simulink model "HyperloopAED"  (R2025b)
settings: Solver=VariableStepAuto  StartTime=0.0  StopTime=30  RelTol=1e-3
settings Model: Creator=PRANAV  LastModifiedBy=PRANAV

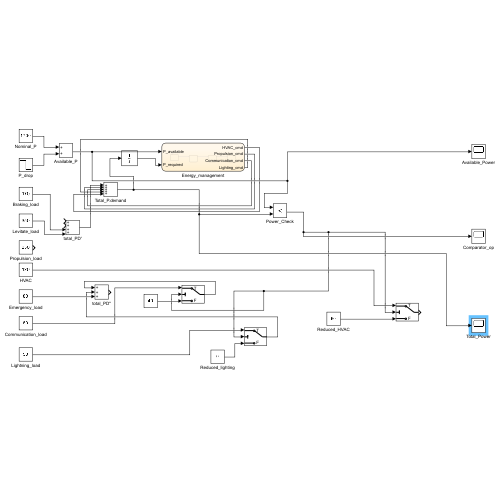
[thumbnail: Simulink's stored preview of the top-level diagram]
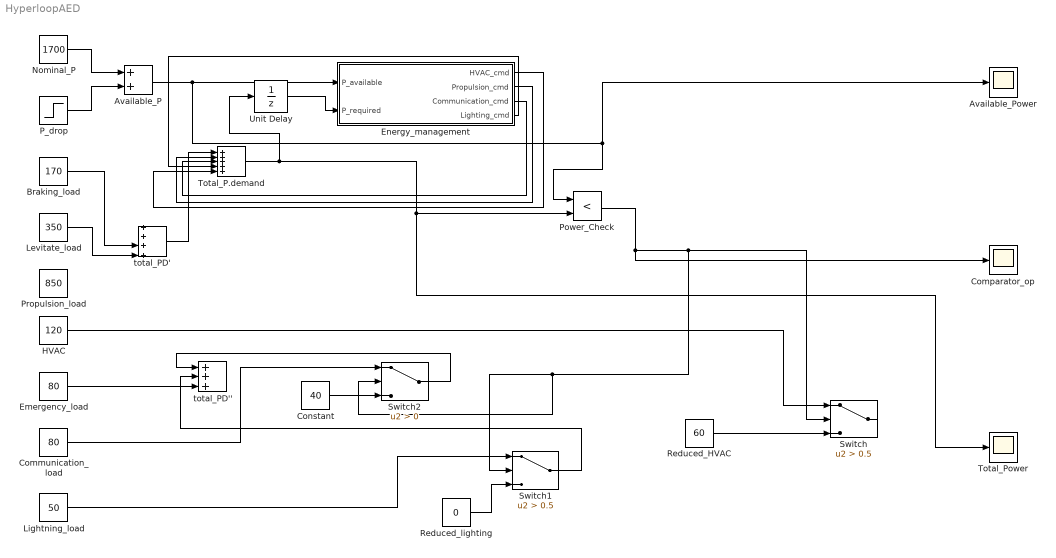
== system HyperloopAED ==
  Available_P : Sum
  Available_Power : Scope
      settings: ActiveDisplayYMinimum=1137.5  ActiveDisplayYMaximum=1762.5
  Braking_load : Constant  Value=170
  Communication_load : Constant  Value=80
  Comparator_op : Scope
      settings: ActiveDisplayYMinimum=-0.12499999999999997  ActiveDisplayYMaximum=1.125
  Constant : Constant  Value=40
  Emergency_load : Constant  Value=80
  Energy_management : Stateflow chart  TreatAsAtomicUnit=on
      settings: PortSchema="{\"entries\":[{\"content\":{\"sides\":[{\"content\":{\"connectorIds\":[\"In1\",\"In2\"]},\"type\":\"ConnectorPlacement.EquallySpacedRectSide\",\"uuid\":\"97038daa-e770-4b03-9197-b8205fec80ee\"},{\"content\":{\"connectorIds\":[\"Out1\",\"Out4\",\"Out3\",\"Out2\"],\"side\":\"RIGHT\"},\"type\":\"ConnectorPlacement.EquallySpacedRectSide\",\"uuid\":\"5d348c5e-e4cd-48d6-bfb1-b7eca039e31a\"},{\"content\":{\"side\":\"TOP\"},\"type\":\"ConnectorPlacement.EquallySpacedRectSide\",\"uuid\":\"902d5b1e-b622-43c9-be24-94d491fd9ea6\"}]},\"type\":\"ConnectorPlacement.EquallySpacedConnector\",\"uuid\":\"16dbb211-ee92-4295-a02a-abd65ddea233\"}],\"packageUris\":[\"http://schema.mathworks.com/mf0/Connector/R2020b\"],\"version\":\"1.0\"}"
  HVAC : Constant  Value=120
  Levitate_load : Constant  Value=350
  Lightning_load : Constant  Value=50
  Nominal_P : Constant  Value=1700
  P_drop : Step  Time=20  After=-500  SampleTime=0
  Power_Check : RelationalOperator  Operator=<  OutDataTypeStr=boolean  RndMeth=Simplest  InputSameDT=off
  Propulsion_load : Constant  Value=850
  Reduced_HVAC : Constant  Value=60
  Reduced_lighting : Constant  Value=0
  Switch : Switch  Criteria=u2 > Threshold  Threshold=0.5  SaturateOnIntegerOverflow=off  InputSameDT=off
  Switch1 : Switch  Criteria=u2 > Threshold  Threshold=0.5  SaturateOnIntegerOverflow=off  InputSameDT=off
  Switch2 : Switch  Criteria=u2 > Threshold  SaturateOnIntegerOverflow=off  InputSameDT=off
  Total_P.demand : Sum  Inputs=+++++
  Total_Power : Scope
      settings: ActiveDisplayYMinimum=965.125219697243  ActiveDisplayYMaximum=2457.5560129704977  DataLoggingVariableName=ScopeData2
  Unit Delay : UnitDelay  InitialCondition=1700  SampleTime=-1  HasFrameUpgradeWarning=on
  total_PD' : Sum  Inputs=++++
  total_PD'' : Sum  Inputs=+++
  wires:
  Nominal_P/1 -> Available_P/1
  P_drop/1 -> Available_P/2
  Levitate_load/1 -> total_PD'/4
  Braking_load/1 -> total_PD'/3
  Emergency_load/1 -> total_PD''/3
  total_PD'/1 -> Total_P.demand/1
  Available_P/1 -> Power_Check/1, Available_Power/1, Energy_management/1(P_available)
  Total_P.demand/1 -> Unit Delay/1, Total_Power/1, Power_Check/2
  Power_Check/1 -> Comparator_op/1, Switch2/2, Switch1/2, Switch/2
  HVAC/1 -> Switch/1
  Reduced_HVAC/1 -> Switch/3
  Lightning_load/1 -> Switch1/1
  Reduced_lighting/1 -> Switch1/3
  Switch1/1 -> total_PD''/2
  Constant/1 -> Switch2/3
  Communication_load/1 -> Switch2/1
  Switch2/1 -> total_PD''/1
  Energy_management/1(HVAC_cmd) -> Total_P.demand/5
  Energy_management/4(Propulsion_cmd) -> Total_P.demand/2
  Energy_management/3(Communication_cmd) -> Total_P.demand/3
  Energy_management/2(Lighting_cmd) -> Total_P.demand/4
  Unit Delay/1 -> Energy_management/2(P_required)

== stateflow chart HyperloopAED/Energy_management ==
  state Normal
    entry:
    HVAC_cmd = 120;
    Lighting_cmd = 50;
    Communication_cmd = 80;
    Propulsion_cmd = 850;
  state mild_def
    entry:
    HVAC_cmd = 60;
    Lighting_cmd = 20;
    Communication_cmd = 60;
    Propulsion_cmd = 700;
  state severe_def
    entry:
    HVAC_cmd = 20;
    Lighting_cmd = 0;
    Communication_cmd = 40;
    Propulsion_cmd = 500;
  state Emergency
    entry:
    HVAC_cmd = 0;
    Lighting_cmd = 0;
    Communication_cmd = 20;
    Propulsion_cmd = 0;
  (default) -> Normal
  Normal -> mild_def : [P_available < 0.95*P_required]
  severe_def -> Emergency : [P_available < 0.5*P_required]
  mild_def -> severe_def : [P_available < 0.8*P_required]
  data: P_available input; P_required input; HVAC_cmd output; Lighting_cmd output; Communication_cmd output; Propulsion_cmd output
